simulink model "PSO_Simulink"  (R2020a)
settings: Solver=FixedStepDiscrete  StartTime=0.0  StopTime=Inf  FixedStep=1  MaxStep=1  MinStep=1  RelTol=1e-3  EnableMultiTasking=on
settings Model: ExtModeTrigDuration=8  Creator=Jason  LastModifiedBy=Jason
settings SolverCC: InitialStep=1  AutoInsertRateTranBlk=on
settings OptimizationCC: DefaultUnderspecifiedDataType=single  EnhancedBackFolding=on  PassReuseOutputArgsAs=Individual arguments  MaxStackSize=1024  OptimizeBlockOrder=speed  DifferentSizesBufferReuse=on  OptimizationCustomize=off  DenormalBehavior=FlushToZero  EfficientTunableParamExpr=on
settings DebuggingCC: ParameterTunabilityLossMsg=error
settings HardwareCC: ProdBitPerChar=16  ProdBitPerInt=16  ProdBitPerPointer=32  ProdBitPerSizeT=32  ProdBitPerPtrDiffT=32  ProdLargestAtomicInteger=Integer  ProdLargestAtomicFloat=None  ProdWordSize=16  ProdLongLongMode=on  ProdHWDeviceType=Texas Instruments->C2000
settings SFSimCC: MATLABDynamicMemAlloc=off
settings RTWCC: SystemTargetFile=ert.tlc  HardwareBoard=TI Delfino F2837xD  TLCOptions=-aInlineSetEventsForThisBaseRateFcn=TLC_FALSE -aSuppressMultiTaskScheduler=TLC_FALSE -aRateBasedStepFcn=1  TemplateMakefile=ert_default_tmf  Toolchain=Texas Instruments Code Composer Studio (C2000)
settings CodeAppCC: ForceParamTrailComments=on  IgnoreCustomStorageClasses=off  OperatorAnnotations=on  SimulinkDataObjDesc=on  SFDataObjDesc=on  InsertBlockDesc=on
settings ERTTargetCC: CodeReplacementLibrary=TI C28x  ExtModeStaticAllocSize=10000

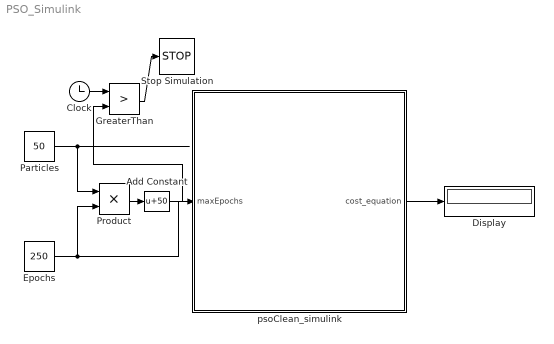
== system PSO_Simulink ==
  Add Constant : Bias  Bias=50
  Clock : Clock
  Display : Display
  Epochs : Constant  Value=250  OutDataTypeStr=single
  GreaterThan : RelationalOperator  Operator=>  OutDataTypeStr=boolean  RndMeth=Simplest
  Particles : Constant  Value=50  OutDataTypeStr=single
  Product : Product
  Stop Simulation : Stop
  psoClean_simulink : MATLAB Function  TreatAsAtomicUnit=on
  wires:
  Clock/1 -> GreaterThan/1
  GreaterThan/1 -> Stop Simulation/1
  Particles/1 -> Product/1
  psoClean_simulink/1(cost_equation) -> Display/1
  Epochs/1 -> psoClean_simulink/1(maxEpochs), Product/2
  Product/1 -> Add Constant/1
  Add Constant/1 -> GreaterThan/2

== matlab function PSO_Simulink/psoClean_simulink ==
  data: cost_equation output; maxEpochs input
function cost_equation  = psoClean(maxEpochs)


persistent currentEpoch currentPar particlesTable neighborIndex EV_bat_n SoC_initial_ev dt Ev_bat_capacity SoC_target_ev Tmax ...
    Tmin T_in_initial V C rho Uwall Uwindow Fwall Fwindow aw Rsej taf_window SC QEC_max QEC_min COP SOC_EV_penalty_multiplier SOC_EV_target_penalty_multiplier ...
    PPEV_diff_penalty_multiplier offset_variable partial_cost_multiplier SoCmax_ev SoCmin_ev lb ub Pmin_ev Pmax_ev Pmax_bat Pmin_bat SoC_initial_bat ...
    SoC_target_bat bat_capacity bat_n span CostOfPower cSelf cSocial inertia outdoor_temperature solar_radiation heatcool_sign Zeta Qin Qsw Qsg U_initial U ...
    QEC_diff_penalty_multiplier Tin_penalty_multiplier T t;

%%%%%%%%%%MALLON LATHOS, FIX LATER
% minNeighborhoodSize = max(2,floor(numParticles*0.25)); %0.25 =Minimum adaptive neighborhood size, a scalar from 0 to 1. Default is 0.25.
minNeighborhoodSize = 2;
%%%%%%%%%%MALLON LATHOS, FIX LATER

numParticles = 50;

numVariables = single(49+25);

tfInvalidMask = single(zeros(numParticles,3*numVariables+1));

%Case: First run of function, initialize variables
if isempty(currentEpoch)
    
    cSelf = single(1.496);
    cSocial = single(1.496);
    %     inertia = 0.798;
    inertia = single(0.398);        %TODO: make inertia vector for each variable
    
    dt=single(0.5);
    T=single(24);
    t = single(0:dt:T);
    
    % CostOfPower(1:14)= 0.07897; CostOfPower(15:46)= 0.11058; CostOfPower(47:49)= 0.07897; %€/kwh
    COP_Ther_Var_struct = load('cop_ther_var.mat');
    COP_Ther_Var=single(COP_Ther_Var_struct.vq1);               %Cost of Power - Summer - Variable
    CostOfPower = COP_Ther_Var;
    
    Pmax_ev = single(5);
    Pmin_ev = single(-5);
    EV_bat_n = single(0.85);
    SoC_initial_ev = single(19.92);
    Ev_bat_capacity = single(35);
    SoC_target_ev = single(20);
    
    Pmax_bat = single(5);
    Pmin_bat = single(-5);
    SoC_initial_bat = single(8);
    SoC_target_bat = single(8);
    bat_capacity = single(15);
    bat_n = single(0.85);
    
    Tmax = single(25);
    Tmin = single(23);
    T_in_initial = single(25);
    V = single(320);
    C = single(1);
    rho = single(1.2);
    Uwall = single(0.00048);
    Uwindow = single(0.0029);
    Fwall = single(224);
    Fwindow = single(20);
    aw = single(18.63);
    Rsej = single(0.04);
    taf_window = single(1.1);
    SC = single(0.54);
    QEC_max = single(5);
    QEC_min = single(0);
    COP = single(3.5);
    solar_radiation_struct = load('solar_radiation.mat');
    outdoor_temperature_struct = load('summer_daily_temperature.mat');
    outdoor_temperature = single(outdoor_temperature_struct.data(1:49));
    solar_radiation = single(solar_radiation_struct.y(1:49));
    heatcool_sign =single(-1);
    
    
    Zeta = single((rho*C*V)/(dt*3600));     %dt is converted to seconds in order to match the rest of the units
    Qin = single(0.2*ones(1,length(t)));
    Qsw = single(aw * Rsej * Uwall * Fwall * solar_radiation);
    Qsg = single(0.001*taf_window * SC * Fwindow * solar_radiation);
    %     Qin = zeros(1,length(t));
    %     Qsw = zeros(1,length(t));
    %     Qsg = zeros(1,length(t));
    
    U = single(((Uwall*Fwall+Uwindow*Fwindow)/Zeta)*outdoor_temperature+(Qin+Qsw+Qsg)/Zeta);
    U_initial=single(((Uwall*Fwall+Uwindow*Fwindow)/Zeta)*outdoor_temperature(1));
    
    
    
    SOC_EV_penalty_multiplier = single(0.05);
    SOC_EV_target_penalty_multiplier = single(1.5);
    PPEV_diff_penalty_multiplier = single(0.05);
    
    QEC_diff_penalty_multiplier = single(0.2);          % Penalty for large deviations of the QEC
    Tin_penalty_multiplier = single(0.6);                 % Penalty for not maintaining the internal temperature between the desired limits
    
    offset_variable = single(4); %Offset the sum of power rates to avoid reaching negative values
    partial_cost_multiplier = single(8);
    
    SoCmax_ev = single(Ev_bat_capacity*0.9);
    SoCmin_ev = single(Ev_bat_capacity*0.1);
    
    lb = single([Pmin_ev*ones(1,49) QEC_min*ones(1,25)]);
    ub = single([Pmax_ev*ones(1,49) QEC_max*ones(1,25)]);
    span = single(ub - lb);
    
    
    currentEpoch = single(0);
    currentPar = single(0);
    particlesTable = single(zeros(numParticles,3*numVariables+1)); %kathe numVariables plithos timon, gia kathe dianusma (current pos, best pos, velocity)
    particlesTable(:,1:numVariables) = repmat(lb,numParticles,1) + repmat(span,numParticles,1) .* rand(numParticles,numVariables);
    particlesTable(:,numVariables+2:numVariables+2+numVariables-1) = particlesTable(:,1:numVariables);
    % Initialize velocities by randomly sampling over the smaller of options.InitialSwarmSpan or ub-lb. Note that min will be InitialSwarmSpan if either lb or ub is not finite.
    vmax = single(span);
    particlesTable(:,2*numVariables+2:2*numVariables+2+numVariables-1) = repmat(-vmax,numParticles,1) + ...
        repmat(2*vmax,numParticles,1) .* rand(numParticles,numVariables);
    
end

%Case: First iteration, initialize variables
if currentEpoch == 0
    
    currentPar = currentPar + 1;
    
    
%     %DEBUG
%     if currentPar == 1
%         rng shuffle;
%     end
    
    
    %% ------------- EV Calculations -------------
    PPEV = single(particlesTable(currentPar,1:49));
    
    PPEV_actual = single(zeros(1,length(PPEV))');
    for z=1:length(PPEV_actual)
        if PPEV(z)>=0
            PPEV_actual(z)=PPEV(z)*EV_bat_n;
        else
            PPEV_actual(z)=PPEV(z)/EV_bat_n;
        end
    end
    
    state_of_charge_ev = single(zeros(1,length(PPEV)));
    state_of_charge_ev(1)=SoC_initial_ev;
    state_of_charge_ev(2:end)=SoC_initial_ev+cumsum(PPEV_actual(1:end-1))*dt;
    
    %% ------------- Heat System Calculations -------------
    QEC_not_interp = single(particlesTable(currentPar,50:74));  % TODO Fix number of variables once you add more power arrays to calculate
    QEC = single(interp1([0:1:24],QEC_not_interp,[0:dt:24],'spline'));
    QEC_thermal = single(QEC*COP);
    
    indoor_temperature=single(zeros(1,length(QEC_thermal)));
    indoor_temperature(1) =T_in_initial;
    
    for i=2:length(QEC)
        indoor_temperature(i) = indoor_temperature(i-1) + heatcool_sign*QEC_thermal(i-1)/Zeta + ...
            (Uwall*Fwall*(outdoor_temperature(i-1)-indoor_temperature(i-1))+ ...
            Uwindow*Fwindow*(outdoor_temperature(i-1)-indoor_temperature(i-1))+ ...
            Qin(i-1)+Qsw(i-1)+Qsg(i-1))/Zeta;
    end
    
    
    %% ------------- EV Penalty -------------
    SOC_ev_penalty = single(0);
    for i=1:length(state_of_charge_ev)
        if state_of_charge_ev(i)>SoCmax_ev
            SOC_ev_penalty = SOC_ev_penalty + (state_of_charge_ev(i) - SoCmax_ev);
        elseif  state_of_charge_ev(i)<SoCmin_ev
            SOC_ev_penalty = SOC_ev_penalty + (SoCmin_ev - state_of_charge_ev(i));
        end
    end
    SOC_ev_target_penalty= single(abs(state_of_charge_ev(end)-SoC_target_ev));
    
    PPEV_diff_penalty = single(sum(abs(diff(PPEV))));
    
    
    %% ------------- Heat System Penalty -------------
    Tin_penalty = single(0);
    for i=1:length(QEC)
        if indoor_temperature(i)>Tmax(1)
            Tin_penalty = Tin_penalty + (indoor_temperature(i) - Tmax(1));
        elseif  indoor_temperature(i)<Tmin(1)
            Tin_penalty = Tin_penalty + (Tmin(1) - indoor_temperature(i));
        end
    end
    QEC_diff_penalty=single(sum(abs(diff(QEC)    )   ));
    
    
    %% ------------- Cost Calculations -------------
    cost_partial = single(sum((PPEV+abs(QEC)).*CostOfPower)*dt);
    cost_equation =single((SOC_EV_target_penalty_multiplier * SOC_ev_target_penalty + SOC_EV_penalty_multiplier * SOC_ev_penalty + ...
        PPEV_diff_penalty_multiplier * PPEV_diff_penalty + QEC_diff_penalty_multiplier*QEC_diff_penalty + Tin_penalty_multiplier*Tin_penalty )+ ...
        (partial_cost_multiplier*(offset_variable+cost_partial)));
    
    particlesTable(currentPar,numVariables+1) = cost_equation; %fval of previous particle stored as the best value of this particle (since it is the first time that it gets a value)
    
    %Finalize initialization
    if currentPar == numParticles
        
        currentEpoch =single(1);
        currentPar = single(0);
    end
    
elseif currentEpoch <= maxEpochs %main loop
    currentPar = currentPar + 1;
    
    if currentPar == 1
        
        % Generate a random neighborhood for each particle that includes the particle itself
        neighborIndex = zeros(numParticles, minNeighborhoodSize);
        neighborIndex(:, 1) = 1:numParticles; % First neighbor is self
        for i = 1:numParticles
            % Determine random neighbors that exclude the particle itself, which is (numParticles-1) particles
            neighbors = randperm(numParticles-1, minNeighborhoodSize-1);
            % Add 1 to indices that are >= current particle index
            iShift = neighbors >= i;
            neighbors(iShift) = neighbors(iShift) + 1;
            neighborIndex(i,2:end) = neighbors;
        end
        
        randSelf = rand(numParticles, numVariables);
        randSocial = rand(numParticles, numVariables);
        
        % Update the velocities
        
        temp1 = inertia*particlesTable(:,2*numVariables+2:2*numVariables+2+numVariables-1);
        temp2 = cSelf*randSelf.*(particlesTable(:,numVariables+2:numVariables+2+numVariables-1)-particlesTable(:,1:numVariables));
        %  temp3 =  cSocial*randSocial.*(particlesTable(bestNeighborIndex,numVariables+2:numVariables+2+numVariables-1)-particlesTable(:,1:numVariables))
        
        temp3 =  cSocial*randSocial.*(particlesTable(neighborIndex(:,2:end),numVariables+2:numVariables+2+numVariables-1)-particlesTable(:,1:numVariables));
        newVelocities =  temp1 + ...
            temp2 + ... %%thesi poy eixe kaluteri timi - current thesi
            temp3;
        
        particlesTable(:,2*numVariables+2:2*numVariables+2+numVariables-1) = newVelocities;
        
        % Update the positions
        newPopulation = particlesTable(:,1:numVariables) + particlesTable(:,2*numVariables+2:2*numVariables+2+numVariables-1);
        
        tfInvalid=zeros(numParticles,numVariables);
        for i=1:numParticles
            tfInvalid(i,:) = newPopulation(i,:) < lb;
        end
        tfInvalidMask(:,2*numVariables+2:end) = tfInvalid;
        mask = (tfInvalidMask==1);
        
        
        if any(any(tfInvalid))
            for y=1:numVariables
                for i=1:numParticles
                    if tfInvalid(i,y)==1
                        newPopulation(i,y)= lb(y);
                    end
                end
            end
            particlesTable(mask) = 0;
        end
        
        
        tfInvalid=zeros(numParticles,numVariables);
        for i=1:numParticles
            tfInvalid(i,:) = newPopulation(i,:) > ub;
        end
        tfInvalidMask(:,2*numVariables+2:end) = tfInvalid;
        mask = (tfInvalidMask==1);
        if any(any(tfInvalid))
            for y=1:numVariables
                for i=1:numParticles
                    if tfInvalid(i,y)==1
                        newPopulation(i,y)= ub(y);
                    end
                end
            end
            particlesTable(mask) = 0;
        end
        particlesTable(:,1:numVariables) = newPopulation;
    end
    
    
    %% ------------- EV Calculations -------------
    PPEV = single(particlesTable(currentPar,1:49));  % TODO Fix number of variables once you add more power arrays to calculate
    
    PPEV_actual = single(zeros(1,length(PPEV))');
    for z=1:length(PPEV_actual)
        if PPEV(z)>=0
            PPEV_actual(z)=PPEV(z)*EV_bat_n;
        else
            PPEV_actual(z)=PPEV(z)/EV_bat_n;
        end
    end
    
    state_of_charge_ev = single(zeros(1,length(PPEV)));
    state_of_charge_ev(1)=SoC_initial_ev;
    state_of_charge_ev(2:end)=SoC_initial_ev+cumsum(PPEV_actual(1:end-1))*dt;
    
    %% ------------- Heat System Calculations -------------
    QEC_not_interp = single(particlesTable(currentPar,50:74));  % TODO Fix number of variables once you add more power arrays to calculate
    QEC = single(interp1([0:1:24],QEC_not_interp,[0:dt:24],'spline'));
    QEC_thermal = single(QEC*COP);
    
    indoor_temperature=single(zeros(1,length(QEC_thermal)));
    indoor_temperature(1) =T_in_initial;
    
    for i=2:length(QEC)
        indoor_temperature(i) = indoor_temperature(i-1) + heatcool_sign*QEC_thermal(i-1)/Zeta + ...
            (Uwall*Fwall*(outdoor_temperature(i-1)-indoor_temperature(i-1))+ ...
            Uwindow*Fwindow*(outdoor_temperature(i-1)-indoor_temperature(i-1))+ ...
            Qin(i-1)+Qsw(i-1)+Qsg(i-1))/Zeta;
    end
    
    %% ------------- EV Penalty -------------
    SOC_ev_penalty = single(0);
    for i=1:length(state_of_charge_ev)
        if state_of_charge_ev(i)>SoCmax_ev
            SOC_ev_penalty = SOC_ev_penalty + (state_of_charge_ev(i) - SoCmax_ev);
        elseif  state_of_charge_ev(i)<SoCmin_ev
            SOC_ev_penalty = SOC_ev_penalty + (SoCmin_ev - state_of_charge_ev(i));
        end
    end
    SOC_ev_target_penalty= single(abs(state_of_charge_ev(end)-SoC_target_ev));
    
    PPEV_diff_penalty = single(sum(abs(diff(PPEV))));
    
    
    %% ------------- Heat System Penalty -------------
    Tin_penalty = single(0);
    for i=1:length(QEC)
        if indoor_temperature(i)>Tmax(1)
            Tin_penalty = Tin_penalty + (indoor_temperature(i) - Tmax(1));
        elseif  indoor_temperature(i)<Tmin(1)
            Tin_penalty = Tin_penalty + (Tmin(1) - indoor_temperature(i));
        end
    end
    QEC_diff_penalty=single(sum(abs(diff(QEC)    )   ));
    
    
    %% ------------- Cost Calculations -------------
    cost_partial = single(sum((PPEV+abs(QEC)).*CostOfPower)*dt);
    
    cost_equation =single((SOC_EV_target_penalty_multiplier * SOC_ev_target_penalty + SOC_EV_penalty_multiplier * SOC_ev_penalty + ...
        PPEV_diff_penalty_multiplier * PPEV_diff_penalty + QEC_diff_penalty_multiplier*QEC_diff_penalty + Tin_penalty_multiplier*Tin_penalty )+ ...
        (partial_cost_multiplier*(offset_variable+cost_partial)));
    
    if cost_equation < particlesTable(currentPar,numVariables+1)
        
        particlesTable(currentPar,numVariables+1) = cost_equation;
        particlesTable(currentPar,numVariables+2:numVariables+2+numVariables-1) = particlesTable(currentPar,1:numVariables);
        
        
    end
    
    if currentPar == numParticles
        
        currentEpoch = currentEpoch + 1;
        currentPar = single(0);
        
        if currentEpoch-1 == maxEpochs
            %DEBUGGING, REMOVE LATER
            [currect_min_cost,~] = min(particlesTable(:,numVariables+1));
            disp(' ')
            disp('Current epoch:')
            disp(currentEpoch-1)
            disp('Current min cost:')
            disp(currect_min_cost)
        end
        
% %           DEBUGGING, REMOVE LATER
%         [currect_min_cost,~] = min(particlesTable(:,numVariables+1));
%         disp(' ')
%         disp('Current epoch:')
%         disp(currentEpoch-1)
%         disp('Current min cost:')
%         disp(currect_min_cost)
        
        return;
        
    elseif currentPar>1 && currentPar<numParticles
        return;
        
    elseif currentPar == 1
        return;
        
    else % never reaches that
        error('Particle Loop Error')
    end
else
    
    [cost_equation,~] = min(particlesTable(:,numVariables+1));
    disp('End of iterations');
    
end
end
